simulink model "ghostfollower"  (R2021a)
settings: Solver=FixedStepAuto  StartTime=0.0  StopTime=inf  FixedStep=0.02  RelTol=1e-3
undefined symbols (not defined in the file): Angular, Linear
libraries: robotlib x16
settings Model: Creator=ivory  LastModifiedBy=refulgent
settings SolverCC: AlgebraicLoopSolver=TrustRegion
settings OptimizationCC: EnhancedBackFolding=on  PassReuseOutputArgsAs=Individual arguments  ZeroExternalMemoryAtStartup=off  ZeroInternalMemoryAtStartup=off  MaxStackSize=64  OptimizeBlockOrder=speed  DifferentSizesBufferReuse=on  OptimizationCustomize=off  EfficientTunableParamExpr=on
settings DebuggingCC: ParameterTunabilityLossMsg=error  SFMachineParentedDataDiag=warning
settings HardwareCC: ProdBitPerPointer=32  ProdBitPerSizeT=32  ProdBitPerPtrDiffT=32  ProdLargestAtomicFloat=None  ProdIntDivRoundTo=Undefined  ProdEndianess=Unspecified  ProdWordSize=32  ProdHWDeviceType=Generic->Unspecified (assume 32-bit Generic)
settings SFSimCC: MATLABDynamicMemAlloc=off  SimTargetLang=C++
settings RTWCC: SystemTargetFile=ert.tlc  HardwareBoard=Robot Operating System (ROS)  TLCOptions="-aInlineSetEventsForThisBaseRateFcn=TLC_FALSE -aSuppressMultiTaskScheduler=TLC_FALSE  -aRateBasedStepFcn=0"  TemplateMakefile=ert_default_tmf  GenerateReport=on  Toolchain=Catkin  IncludeHyperlinkInReport=on  LaunchReport=on  TargetLang=C++  GenerateTraceInfo=on  GenerateTraceReport=on  GenerateTraceReportSl=on  GenerateTraceReportSf=on  GenerateTraceReportEml=on
settings CodeAppCC: ForceParamTrailComments=on  IgnoreCustomStorageClasses=off  OperatorAnnotations=on  SimulinkDataObjDesc=on  SFDataObjDesc=on  InsertBlockDesc=on
settings ERTTargetCC: SupportContinuousTime=on  SupportVariableSizeSignals=on

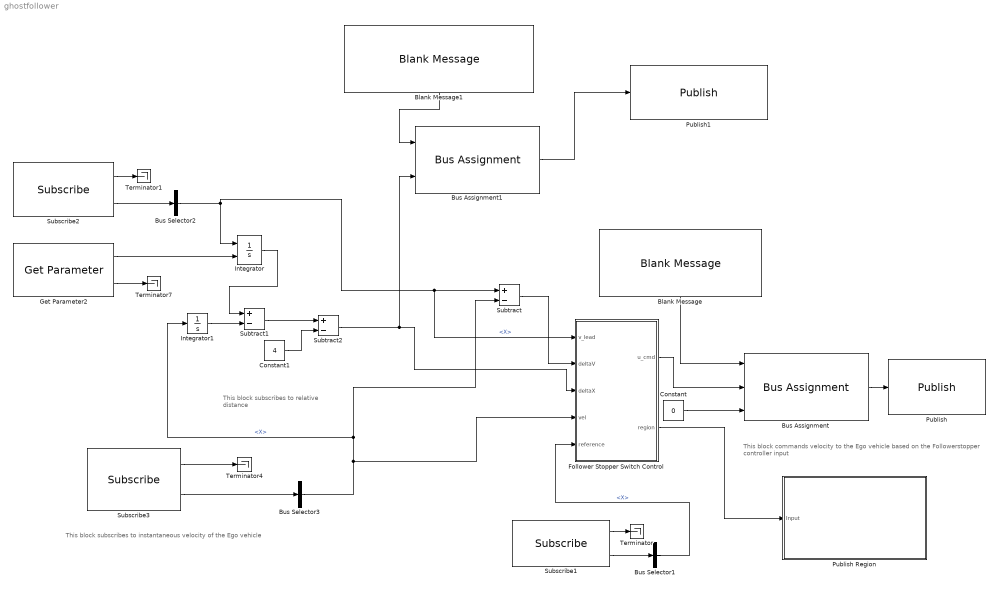
== system ghostfollower ==
  note: This block subscribes to
      | instantaneous velocity of the Ego vehicle
  note: This block subscribes
      | to relative distance
  note: This block commands velocity to the Ego vehicle based
      | on the Followerstopper controller input
  Blank Message : robotlib/Blank Message  messageClass=Message  entityType=geometry_msgs/Twist  messageType=geometry_msgs/Twist  SampleTime=inf  legacyBusStruct=off
  Blank Message1 : robotlib/Blank Message  messageClass=Message  entityType=std_msgs/Float64  messageType=std_msgs/Float64  SampleTime=inf  legacyBusStruct=off
  Bus Assignment : BusAssignment  AssignedSignals=Linear.X,Angular.Z
  Bus Assignment1 : BusAssignment  AssignedSignals=Data
  Bus Selector1 : BusSelector  OutputSignals=Linear.X
  Bus Selector2 : BusSelector  OutputSignals=Linear.X
  Bus Selector3 : BusSelector  OutputSignals=Linear.X
  Constant : Constant  Value=0
  Constant1 : Constant  Value=4
  Follower Stopper Switch Control : Subsystem
  Get Parameter2 : robotlib/Get Parameter  ParameterSource=Specify your own  ParameterName=init_gap  ParameterType=double  ParameterMaxArrayLength=16  ParameterInitialValue=30.0  SampleTime=-1  ShowErrorCodeOutput=on  ModelName=ghostfollower  BlockId=ParamGet_ghostfollower_236
      settings: SourceProductBaseCode=RR
  Integrator : Integrator  InitialConditionSource=external
  Integrator1 : Integrator
  Publish : robotlib/Publish  topicSource=Specify your own  topic=cmd_vel  messageType=geometry_msgs/Twist  legacyBusStruct=off  messageQueueLength=1
  Publish Region : Subsystem
  Publish1 : robotlib/Publish  topicSource=Specify your own  topic=headway_est  messageType=std_msgs/Float64  legacyBusStruct=off  messageQueueLength=1
  Subscribe1 : robotlib/Subscribe  topicSource=Specify your own  topic=v_ref  messageType=geometry_msgs/Twist  SampleTime=-1  legacyBusStruct=off  messageQueueLength=1
  Subscribe2 : robotlib/Subscribe  topicSource=Specify your own  topic=leader_vel  messageType=geometry_msgs/Twist  SampleTime=-1  legacyBusStruct=off  messageQueueLength=1
  Subscribe3 : robotlib/Subscribe  topicSource=Specify your own  topic=vel  messageType=geometry_msgs/Twist  SampleTime=-1  legacyBusStruct=off  messageQueueLength=1
  Subtract : Sum  Inputs=+-
  Subtract1 : Sum  Inputs=+-
  Subtract2 : Sum  Inputs=+-
  Terminator{,1,4,7} (4 alike) : Terminator
  wires:
  Bus Assignment/1 -> Publish/1
  Subscribe3/2 -> Bus Selector3/1
  Blank Message/1 -> Bus Assignment/1
  Bus Selector3/1 -> Subtract/2, Integrator1/1, Follower Stopper Switch Control/4(vel)  "<X>"
  Constant/1 -> Bus Assignment/3
  Subscribe3/1 -> Terminator4/1
  Follower Stopper Switch Control/1(u_cmd) -> Bus Assignment/2
  Bus Selector1/1 -> Follower Stopper Switch Control/5(reference)  "<X>"
  Follower Stopper Switch Control/2(region) -> Publish Region/1(Input)
  Subscribe1/1 -> Terminator/1
  Subscribe1/2 -> Bus Selector1/1
  Subscribe2/2 -> Bus Selector2/1
  Bus Selector2/1 -> Follower Stopper Switch Control/1(v_lead), Subtract/1, Integrator/1  "<X>"
  Subscribe2/1 -> Terminator1/1
  Get Parameter2/2 -> Terminator7/1
  Get Parameter2/1 -> Integrator/2
  Subtract/1 -> Follower Stopper Switch Control/2(deltaV)
  Bus Assignment1/1 -> Publish1/1
  Subtract2/1 -> Follower Stopper Switch Control/3(deltaX), Bus Assignment1/2
  Blank Message1/1 -> Bus Assignment1/1
  Constant1/1 -> Subtract2/2
  Subtract1/1 -> Subtract2/1
  Integrator/1 -> Subtract1/1
  Integrator1/1 -> Subtract1/2

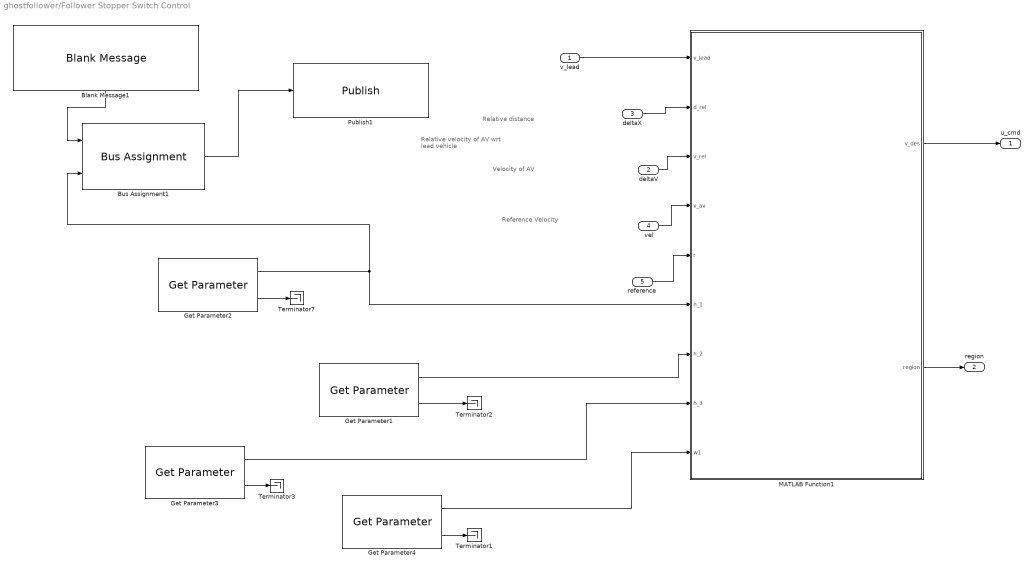
== system ghostfollower/Follower Stopper Switch Control ==
  note: Relative velocity of
      | AV wrt lead vehicle
  note: Velocity of AV
  note: Reference Velocity
  note: Relative distance
  v_lead : Inport
  deltaV : Inport  Port=2
  deltaX : Inport  Port=3
  vel : Inport  Port=4
  reference : Inport  Port=5
  Blank Message1 : robotlib/Blank Message  messageClass=Message  entityType=std_msgs/Float64  messageType=std_msgs/Float64  SampleTime=inf  legacyBusStruct=off
  Bus Assignment1 : BusAssignment  AssignedSignals=Data
  Get Parameter1 : robotlib/Get Parameter  ParameterSource=Specify your own  ParameterName=th2  ParameterType=double  ParameterMaxArrayLength=16  ParameterInitialValue=1.2  SampleTime=-1  ShowErrorCodeOutput=on  ModelName=ghostfollower  BlockId=ParamGet_ghostfollower_228
      settings: SourceProductBaseCode=RR
  Get Parameter2 : robotlib/Get Parameter  ParameterSource=Specify your own  ParameterName=th1  ParameterType=double  ParameterMaxArrayLength=16  ParameterInitialValue=0.4  SampleTime=-1  ShowErrorCodeOutput=on  ModelName=ghostfollower  BlockId=ParamGet_ghostfollower_226
      settings: SourceProductBaseCode=RR
  Get Parameter3 : robotlib/Get Parameter  ParameterSource=Specify your own  ParameterName=th3  ParameterType=double  ParameterMaxArrayLength=16  ParameterInitialValue=1.8  SampleTime=-1  ShowErrorCodeOutput=on  ModelName=ghostfollower  BlockId=ParamGet_ghostfollower_230
      settings: SourceProductBaseCode=RR
  Get Parameter4 : robotlib/Get Parameter  ParameterSource=Specify your own  ParameterName=w1  ParameterType=double  ParameterMaxArrayLength=16  ParameterInitialValue=4.5  SampleTime=-1  ShowErrorCodeOutput=on  ModelName=ghostfollower  BlockId=ParamGet_ghostfollower_245
      settings: SourceProductBaseCode=RR
  MATLAB Function1 : MATLAB Function  TreatAsAtomicUnit=on
  Publish1 : robotlib/Publish  topicSource=Specify your own  topic=timheadway1  messageType=std_msgs/Float64  legacyBusStruct=off  messageQueueLength=1
  Terminator{1..3,7} (4 alike) : Terminator
  u_cmd : Outport
  region : Outport  Port=2
  wires:
  deltaX/1 -> MATLAB Function1/2(d_rel)
  deltaV/1 -> MATLAB Function1/3(v_rel)
  vel/1 -> MATLAB Function1/4(v_av)
  v_lead/1 -> MATLAB Function1/1(v_lead)
  reference/1 -> MATLAB Function1/5(r)
  MATLAB Function1/1(v_des) -> u_cmd/1
  MATLAB Function1/2(region) -> region/1
  Get Parameter3/1 -> MATLAB Function1/8(h_3)
  Get Parameter1/2 -> Terminator2/1
  Get Parameter1/1 -> MATLAB Function1/7(h_2)
  Get Parameter3/2 -> Terminator3/1
  Get Parameter2/2 -> Terminator7/1
  Blank Message1/1 -> Bus Assignment1/1
  Bus Assignment1/1 -> Publish1/1
  Get Parameter2/1 -> Bus Assignment1/2, MATLAB Function1/6(h_1)
  Get Parameter4/2 -> Terminator1/1
  Get Parameter4/1 -> MATLAB Function1/9(w1)

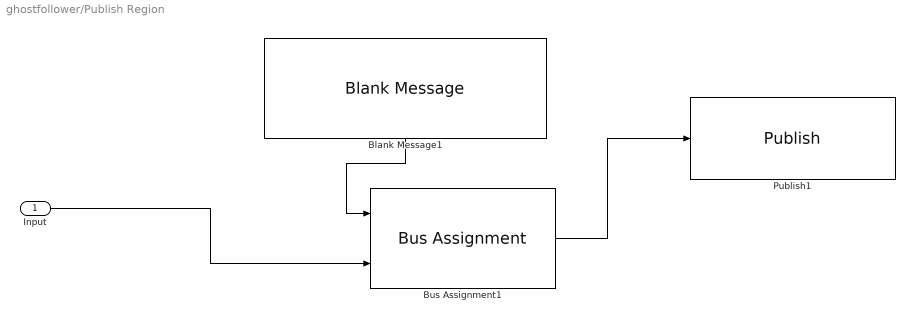
== system ghostfollower/Publish Region ==
  Input : Inport
  Blank Message1 : robotlib/Blank Message  messageClass=Message  entityType=std_msgs/UInt8  messageType=std_msgs/UInt8  SampleTime=inf  legacyBusStruct=off
  Bus Assignment1 : BusAssignment  AssignedSignals=Data
  Publish1 : robotlib/Publish  topicSource=Specify your own  topic=region  messageType=std_msgs/UInt8  legacyBusStruct=off  messageQueueLength=1
  wires:
  Input/1 -> Bus Assignment1/2
  Blank Message1/1 -> Bus Assignment1/1
  Bus Assignment1/1 -> Publish1/1

== matlab function ghostfollower/Follower Stopper Switch Control/MATLAB Function1 ==
  data: v_lead input; v_des output; d_rel input; v_rel input; v_av input; r input; region output; h_1 input; h_2 input; h_3 input; w1 input
function [v_des, region]= fcn(v_lead, d_rel,v_rel,v_av, r, h_1, h_2, h_3, w1)
%#codegen
% Safety controller, based on quadratic bands.
% Input: r = desired velocity (from other models)
%          d_rel = estimate of gap to vehicle ahead
%          v_rel = estimate of time derivative of dx (= velocity difference)
%         v_AV = velocity of AV
%      dx_min = minimum distance
% dx_activate = distance below which controller does something
%       decel = vector of three deceleration values for parabolas
% Out:  u_cmd = actual velocity commanded (always u_cmd<=U)
%
% Controller-specific parameters

    w = zeros(3,1);
    alpha = zeros(3,1);
    w(1) = w1;
    alpha(1) = 1.5;
    w(3) = 6.0;
    alpha(3) = 0.5;
    w(2) = (w(1)+w(3))/2;
    alpha(2) = (alpha(1)+alpha(3))/2;
    if(nargin<4)
        r = 30;
    end
    
    %v_rel_star = min(v_rel,0)
    v_rel_star = v_rel;
    v_rel_star(v_rel >= 0) = 0;
    
%     h_1 = 0.4;
%     h_2 = 1.2;
%     h_3 = 1.8;
    
    x1 = w(1) + (0.5*v_rel_star.^2)/alpha(1) + h_1*v_av;
    x2 = w(2) + (0.5*v_rel_star.^2)/alpha(2) + h_2*v_av;
    x3 = w(3) + (0.5*v_rel_star.^2)/alpha(3) + h_3*v_av;
    
%     v_lead = v_av+v_rel;
    
    
    %v = min([max([v_lead,0]),r]);
    v = v_lead;
    v(v_lead<0) = 0;
    
    v(v_lead>r) = r;
  
    v_des = zeros(size(d_rel)); 
    %safe region
    v_des(d_rel>x3) = r;  
    %adaptation region 2
    temp_v_des = v+(r-v).*(d_rel-x2)./(x3-x2);
    v_des(d_rel>x2 & d_rel<=x3) = temp_v_des(d_rel>x2 & d_rel<=x3);   
    %adaptation region 1
    temp_v_des = v.*(d_rel-x1)./(x2-x1);
    v_des(d_rel>x1 & d_rel<=x2) = temp_v_des(d_rel>x1 & d_rel<=x2); 
    
    if d_rel>x3
        region = uint8(0);
    elseif d_rel>x2 && d_rel<=x3
        region = uint8(1);
    elseif d_rel>x1 && d_rel<=x2
        region = uint8(2);
    else
        region = uint8(3);
    end
